simulink model "irep_single_axis"  (Simulink 7.5)
settings: Solver=ode3  StartTime=0.0  StopTime=inf  FixedStep=dt  RelTol=1e-3
InitFcn:
  | IREPOLD_DEPENDENCY
  | init_omni
  | init_filters
  | init_invivo
  | init_telemanipulation
  | init_parker_xyz
  | init_magnetic_tracker
  | init_loadcell
  | init_scopes
  | init_homing
  | init_force_control
  | ATI_Init_nano17
undefined symbols (not defined in the file): A, ATI_torque_convert_to_Nmm, counter_offset, DiscIntNeverNeededParam, dt, encoder_counts, filter_coeffs_ATI, filter_coeffs_ATI_bias, gear_ratio, HomingFineEps, HomingRoughEps, HomingRoughVelocity, inv_T, joystick_filter_coeffs, K_d, K_i, K_p, left_arm_home_voltage, N_ATI, N_ATI_bias, N_joystick, N_pots, pots_filter_coeffs, quadrature_mode, right_arm_home_voltage, RightArmHomingDirectionVector, RightArmHomingIntGain, screw_pitch
libraries: xpcconteclib x23, xpcmeasurementcomputinglib x17, xpclib x11, simulink x8, dspswit3 x4, dspsigops x1, powerlib_extras x1
(part 1 of 3)
settings Model: Creator=Andrea  LastModifiedBy=Long  BufferReuse=off
settings OptimizationCC: BlockReduction=off  OptimizeBlockIOStorage=off  BufferReuse=off  ExpressionFolding=off  LocalBlockOutputs=off  OptimizeModelRefInitCode=on
settings DebuggingCC: MultiTaskCondExecSysMsg=warning  MultiTaskRateTransMsg=warning  StrictBusMsg=Warning
settings HardwareCC: ProdIntDivRoundTo=Zero  ProdEndianess=LittleEndian  ProdHWDeviceType=Generic->32-bit x86 compatible
settings RTWCC: SystemTargetFile=xpctargetert.tlc  TemplateMakefile=xpc_ert_tmf  Description=xPC Target (ERT)  ProcessScript=xpctargetert_make_rtw_hook  RTWCompilerOptimization=On
settings xpcTargetERTCC: TargetFcnLib=ansi_tfl_table_tmw.mat  TargetFunctionLibrary=ANSI_C  UtilityFuncGeneration=Auto  ERTMultiwordTypeDef=System defined  ERTCodeCoverageTool=None  ERTMultiwordLength=256  MultiwordLength=2048  GenerateFullHeader=on  GenerateSampleERTMain=off  GenerateTestInterfaces=off  IsPILTarget=off  ModelReferenceCompliant=on  ParMdlRefBuildCompliant=off  CompOptLevelCompliant=on  IncludeMdlTerminateFcn=on  GeneratePreprocessorConditionals=Disable all  CombineOutputUpdateFcns=off  SuppressErrorStatus=off  ERTFirstTimeCompliant=off  IncludeFileDelimiter=Auto  ERTCustomFileBanners=off  SupportAbsoluteTime=on  LogVarNameModifier=rt_  MatFileLogging=on  MultiInstanceERTCode=off  SupportNonFinite=on  SupportComplex=on  PurelyIntegerCode=off  SupportContinuousTime=on  SupportNonInlinedSFcns=on  SupportVariableSizeSignals=off  EnableShiftOperators=on  ParenthesesLevel=Nominal  PortableWordSizes=off  ModelStepFunctionPrototypeControlCompliant=off  CPPClassGenCompliant=off  AutosarCompliant=off  GenerateASAP2=off  ExtModeTransport=0  ExtModeStaticAlloc=off  ExtModeStaticAllocSize=1000000  ExtModeTesting=off  InlinedParameterPlacement=NonHierarchical  TargetOS=BareBoardExample  MultiInstanceErrorCode=Error  RateGroupingCode=on  RootIOFormat=Individual arguments  CoverageDialogOpen=off  ERTFilePackagingFormat=Modular  PreserveExpressionOrder=off  PreserveIfCondition=off  ConvertIfToSwitch=off  PreserveExternInFcnDecls=on  EnableUserReplacementTypes=off  MemSecPackage=--- None ---  MemSecDataConstants=Default  MemSecDataIO=Default  MemSecDataInternal=Default  MemSecDataParameters=Default  MemSecFuncInitTerm=Default  MemSecFuncExecute=Default  GRTInterface=on  GlobalDataDefinition=Auto  GlobalDataReference=Auto  ModuleNamingRule=Unspecified  ERTSrcFileBannerTemplate=ert_code_template.cgt  ERTHdrFileBannerTemplate=ert_code_template.cgt  ERTDataSrcFileTemplate=ert_code_template.cgt  ERTDataHdrFileTemplate=ert_code_template.cgt  ERTCustomFileTemplate=example_file_process.tlc  SignalDisplayLevel=10  ParamTuneLevel=10  InitialValueSource=Model  RTWCAPISignals=off  RTWCAPIParams=off  RTWCAPIStates=off  GenerateErtSFunction=off  RL32ModeModifier=Real-Time  ExtMode=on  ExtModeMexFile=ext_xpc  ExtModeIntrfLevel=Level2 - Open  ExtModeArmWhenConnect=off  RL32LogTETModifier=on  RL32LogBufSizeModifier=100000  RL32IRQSourceModifier=Timer  xPCIRQSourceBoard=None/Other  xPCIOIRQSlot=-1  xpcObjCom=off  xPCGenerateASAP2=off  xPCGenerateXML=off  RL32ObjectName=tg  xPCisDownloadable=off  xPCisDefaultEnv=on  xPCisModelTimeout=on  xPCModelTimeoutSecs=5  xpcDblBuff=off  xPCLoadParamSetFile=off

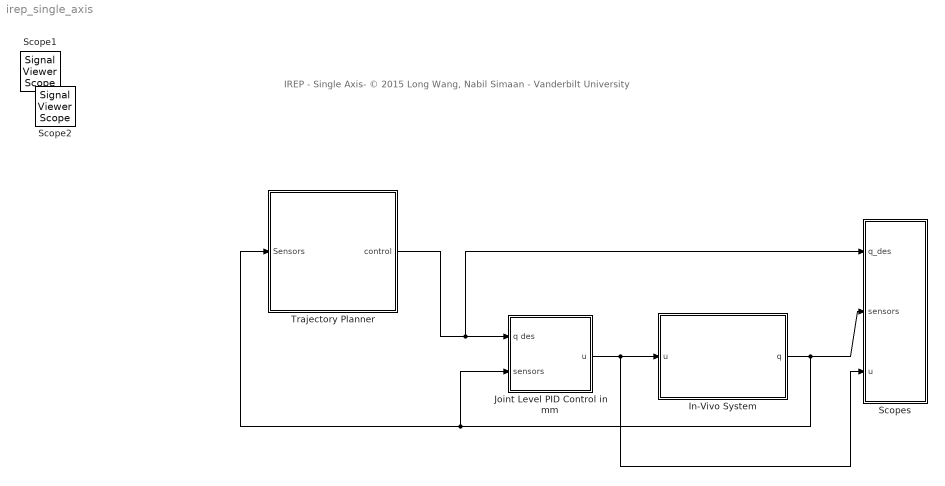
== system irep_single_axis ==
  note: IREP - Single Axis- © 2015 Long Wang, Nabil Simaan - Vanderbilt University
  In-Vivo System : Subsystem
      mask Display: image(imread('irep.png'));
  Joint Level PID Control in mm : Subsystem
  Scopes : Subsystem
  Trajectory Planner : Subsystem
  Scope1 : SignalViewerScope  IOType=viewer  RefreshTime=0.035000
  Scope2 : SignalViewerScope  IOType=viewer  RefreshTime=0.035000
  wires:
  In-Vivo System/1(q) -> Joint Level PID Control in mm/2(sensors), Trajectory Planner/1(Sensors), Scopes/2(sensors)
  Joint Level PID Control in mm/1(u) -> In-Vivo System/1(u), Scopes/3(u)
  Trajectory Planner/1(control) -> Joint Level PID Control in mm/1(q des), Scopes/1(q_des)

== system irep_single_axis/In-Vivo System ==
  u : Inport  OutDataType=fixdt(1, 16)  OutScaling=2^0
  ATI FT Sensor : Subsystem
  ATI FT Sensor enable : Constant  Value=0  OutDataType=fixdt(1, 16)  OutScaling=2^0
  Bus Creator : BusCreator  Inputs=5
  CONTEC CARDS : Subsystem
  Count to mm : Subsystem
  D/A : Subsystem
  Digital_Inputs : Subsystem
  Motor Enable : Subsystem
  Potentiometers : Subsystem
  q : Outport
  wires:
  CONTEC CARDS/1(Out1) -> Count to mm/1(counts)
  u/1 -> D/A/1(In1)
  Potentiometers/1(Pots) -> Bus Creator/2  "A/D signals"
  Bus Creator/1 -> q/1
  Count to mm/1(q_cur_system) -> Bus Creator/1  "q"
  Digital_Inputs/1(foot switches) -> Bus Creator/3  "foot switches"
  Digital_Inputs/2(Pot_connect) -> Bus Creator/4  "Pots_Connect"
  ATI FT Sensor/1(Forces) -> Bus Creator/5  "ATI"
  ATI FT Sensor enable/1 -> ATI FT Sensor/Enable

== system irep_single_axis/Joint Level PID Control in mm ==
  q des : Inport  OutDataType=fixdt(1, 16)  OutScaling=2^0
  sensors : Inport  Port=2  OutDataType=fixdt(1, 16)  OutScaling=2^0
  Bus Creator : Subsystem
  Bus selector : Subsystem
  Enable Control : Constant  Value=0  OutDataType=fixdt(1, 16)  OutScaling=2^0
  PID Compensator : Subsystem
  Sum : Sum  Inputs=|+-  OutDataType=fixdt(1, 16)  OutScaling=2^0  SampleTime=dt
  u : Outport  OutDataType=fixdt(1, 16)  OutScaling=2^0
  wires:
  q des/1 -> Sum/1
  Sum/1 -> PID Compensator/1(e)
  sensors/1 -> Bus selector/1(sensors)
  Bus selector/1(Out1) -> Sum/2
  PID Compensator/1(u) -> Bus Creator/1(In1)
  Bus Creator/1(Out1) -> u/1
  Enable Control/1 -> PID Compensator/Enable

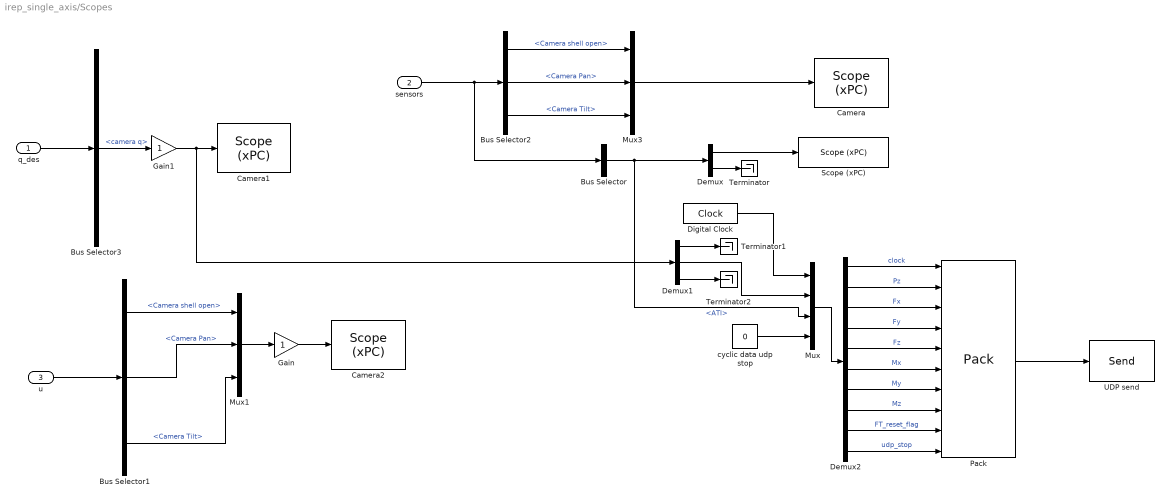
== system irep_single_axis/Scopes ==
  q_des : Inport
  sensors : Inport  Port=2
  u : Inport  Port=3
  Bus Selector : BusSelector  OutputSignals=ATI
  Bus Selector1 : BusSelector  OutputSignals=Camera shell open,Camera Pan,Camera Tilt
  Bus Selector2 : BusSelector  OutputSignals=q.Camera shell open,q.Camera Pan,q.Camera Tilt
  Bus Selector3 : BusSelector  OutputSignals=camera q
  Camera : xpclib/Misc./Scope (xPC)   SystemSampleTime=-1  scopeno=1  scopetype=Target  autostart=on  viewmode=Numerical  formatstr='Camera cur: %3.3f'  grid=on  ylimits=[0,0]  nosamples=10  noprepostsamples=0  interleave=1  triggermode=FreeRun  triggersignal=1  triggerlevel=0.0  triggerslope=Either  triggerscope=1  triggersample=0  filename=weights1.dat  mode=Lazy  writesize=512  autorestart=off  dynamicfilemode=off  maxwritefilesize=512*1024^2
  Camera1 : xpclib/Misc./Scope (xPC)   SystemSampleTime=-1  scopeno=2  scopetype=Target  autostart=on  viewmode=Numerical  formatstr='Camera des: %3.3f'  grid=on  ylimits=[0,0]  nosamples=10  noprepostsamples=0  interleave=1  triggermode=FreeRun  triggersignal=1  triggerlevel=0.0  triggerslope=Either  triggerscope=1  triggersample=0  filename=weights1.dat  mode=Lazy  writesize=512  autorestart=off  dynamicfilemode=off  maxwritefilesize=512*1024^2
  Camera2 : xpclib/Misc./Scope (xPC)   SystemSampleTime=-1  scopeno=3  scopetype=Target  autostart=on  viewmode=Numerical  formatstr='Camera u: %3.3f'  grid=on  ylimits=[0,0]  nosamples=10  noprepostsamples=0  interleave=1  triggermode=FreeRun  triggersignal=1  triggerlevel=0.0  triggerslope=Either  triggerscope=1  triggersample=0  filename=weights1.dat  mode=Lazy  writesize=512  autorestart=off  dynamicfilemode=off  maxwritefilesize=512*1024^2
  Demux : Demux  Outputs=[6,1]
  Demux1 : Demux  Outputs=3
  Demux2 : Demux  Outputs=10
  Digital Clock : DigitalClock  SampleTime=dt
  Gain : Gain  ParameterDataType=fixdt(1, 16)  ParameterScaling=2^0  OutDataType=fixdt(1, 16)  OutScaling=2^0
  Gain1 : Gain  ParameterDataType=fixdt(1, 16)  ParameterScaling=2^0  OutDataType=fixdt(1, 16)  OutScaling=2^0
  Mux : Mux
  Mux1 : Mux  Inputs=3
  Mux3 : Mux  Inputs=3
  "Pack " : xpclib/UDP/Pack  datatypes={'double' 'double' 'double' 'double' 'double' 'double' 'double' 'double' 'double' 'double'}  byteAlign=1
  "Scope (xPC) " : xpclib/Misc./Scope (xPC)   SystemSampleTime=-1  scopeno=20  scopetype=Target  autostart=on  viewmode=Numerical  formatstr=scope_format_ATI_wrench  grid=on  ylimits=[0,0]  nosamples=25  noprepostsamples=0  interleave=1  triggermode=FreeRun  triggersignal=1  triggerlevel=0.0  triggerslope=Either  triggerscope=1  triggersample=0  filename=data.dat  mode=Lazy  writesize=512  autorestart=off  dynamicfilemode=off  maxwritefilesize=512*1024^2
  Terminator : Terminator
  Terminator1 : Terminator
  Terminator2 : Terminator
  UDP send : xpclib/UDP/Send  ipAddress=192.168.1.101  ipPort=25001  localPort=-1  vblLen=off  sampletime=0.008
  cyclic data udp stop : Constant  Value=0  OutDataType=fixdt(1, 16)  OutScaling=2^0
  wires:
  sensors/1 -> Bus Selector/1, Bus Selector2/1
  q_des/1 -> Bus Selector3/1
  Bus Selector3/1 -> Gain1/1  "<camera q>"
  Mux3/1 -> Camera/1
  Bus Selector2/1 -> Mux3/1  "<Camera shell open>"
  Bus Selector2/2 -> Mux3/2  "<Camera Pan>"
  Bus Selector2/3 -> Mux3/3  "<Camera Tilt>"
  u/1 -> Bus Selector1/1
  Bus Selector1/1 -> Mux1/1  "<Camera shell open>"
  Bus Selector1/2 -> Mux1/2  "<Camera Pan>"
  Bus Selector1/3 -> Mux1/3  "<Camera Tilt>"
  Mux1/1 -> Gain/1
  Gain/1 -> Camera2/1
  Gain1/1 -> Camera1/1, Demux1/1
  Bus Selector/1 -> Demux/1, Mux/3  "<ATI>"
  Demux/1 -> "Scope (xPC) "/1
  Demux/2 -> Terminator/1
  Demux1/1 -> Terminator1/1
  Demux1/3 -> Terminator2/1
  Digital Clock/1 -> Mux/1
  Demux1/2 -> Mux/2
  Mux/1 -> Demux2/1
  Demux2/1 -> "Pack "/1  "clock"
  Demux2/2 -> "Pack "/2  "Pz"
  Demux2/3 -> "Pack "/3  "Fx"
  Demux2/4 -> "Pack "/4  "Fy"
  Demux2/5 -> "Pack "/5  "Fz"
  Demux2/6 -> "Pack "/6  "Mx"
  Demux2/7 -> "Pack "/7  "My"
  Demux2/8 -> "Pack "/8  "Mz"
  Demux2/9 -> "Pack "/9  "FT_reset_flag"
  "Pack "/1 -> UDP send/1
  cyclic data udp stop/1 -> Mux/4
  Demux2/10 -> "Pack "/10  "udp_stop"

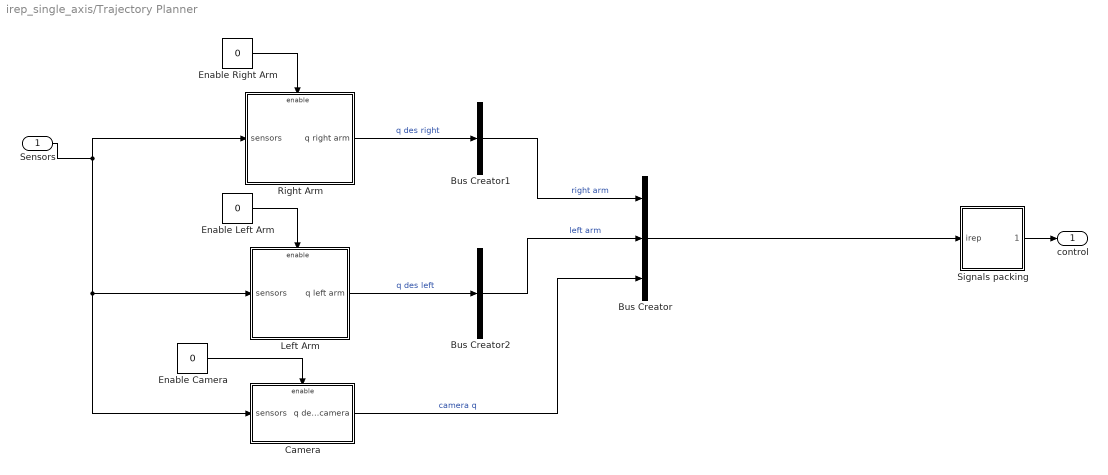
== system irep_single_axis/Trajectory Planner ==
  Sensors : Inport
  Bus Creator : BusCreator  Inputs=3
  Bus Creator1 : BusCreator  Inputs=1
  Bus Creator2 : BusCreator  Inputs=1
  Camera : Subsystem  TreatAsAtomicUnit=on
  Enable Camera : Constant  Value=0  OutDataType=fixdt(1, 16)  OutScaling=2^0  SampleTime=dt
  Enable Left Arm : Constant  Value=0  OutDataType=fixdt(1, 16)  OutScaling=2^0  SampleTime=dt
  Enable Right Arm : Constant  Value=0  OutDataType=fixdt(1, 16)  OutScaling=2^0  SampleTime=dt
  Left Arm : Subsystem  TreatAsAtomicUnit=on
  Right Arm : Subsystem  TreatAsAtomicUnit=on
  Signals packing : Subsystem
  control : Outport  PortDimensions=[23 1]  SampleTime=dt
  wires:
  Enable Right Arm/1 -> Right Arm/Enable
  Enable Left Arm/1 -> Left Arm/Enable
  Enable Camera/1 -> Camera/Enable
  Signals packing/1(system) -> control/1
  Sensors/1 -> Right Arm/1(sensors), Left Arm/1(sensors), Camera/1(sensors)
  Right Arm/1(q right arm) -> Bus Creator1/1  "q des right"
  Bus Creator1/1 -> Bus Creator/1  "right arm"
  Bus Creator2/1 -> Bus Creator/2  "left arm"
  Camera/1(q des camera) -> Bus Creator/3  "camera q"
  Bus Creator/1 -> Signals packing/1(irep)
  Left Arm/1(q left arm) -> Bus Creator2/1  "q des left"

== system irep_single_axis/In-Vivo System/ATI FT Sensor ==
  Enable : EnablePort
  ATI FT Sensor - 20001 : xpclib/UDP/Receive  ipAddress=0.0.0.0  ipPort=20001  width=48  vblLen=on  sampletime=2*dt
  ATI Force Torque Sensor : Subsystem
  Demux : Demux  Outputs=6
  Multiport Switch : MultiPortSwitch  DataPortOrder=Zero-based contiguous  Inputs=2  zeroidx=on  OutDataType=fixdt(1, 16)  OutScaling=2^0
  Mux : Mux  Inputs=7
  Mux1 : Mux  Inputs=6
  Rate Transition : RateTransition  OutPortSampleTime=dt
  Terminator1 : Terminator
  Unpack 2 : xpclib/UDP/Unpack  dimensions={1,1,1,1,1,1}  datatypes={'double' 'double' 'double' 'double' 'double' 'double'}  byteAlign=1
  input source : Constant  OutDataType=fixdt(1, 16)  OutScaling=2^0
  Forces : Outport
  wires:
  ATI FT Sensor - 20001/1 -> Unpack 2/1
  ATI FT Sensor - 20001/2 -> Terminator1/1
  Unpack 2/2 -> Mux1/2  "Fy"
  Unpack 2/3 -> Mux1/3  "Fz"
  Unpack 2/4 -> Mux1/4  "Mx"
  Unpack 2/5 -> Mux1/5  "My"
  Unpack 2/6 -> Mux1/6  "Mz"
  Unpack 2/1 -> Mux1/1  "Fx"
  Mux1/1 -> Rate Transition/1
  ATI Force Torque Sensor/1(wrench) -> Multiport Switch/3
  input source/1 -> Multiport Switch/1
  Demux/1 -> Mux/1  "Fx"
  Demux/2 -> Mux/2  "Fy"
  Demux/3 -> Mux/3  "Fz"
  Demux/4 -> Mux/4  "Mx"
  Demux/5 -> Mux/5  "My"
  Demux/6 -> Mux/6  "Mz"
  Multiport Switch/1 -> Demux/1
  Mux/1 -> Forces/1
  Rate Transition/1 -> Multiport Switch/2
  ATI Force Torque Sensor/2(reset flag) -> Mux/7  "FT_Reset_Flag"

== system irep_single_axis/In-Vivo System/CONTEC CARDS ==
  Level 1 : Subsystem
  Level 2 : Subsystem
  Level 3 : Subsystem
  Mux : Mux
  RZ : Subsystem
  Out1 : Outport
  wires:
  Level 1/1(Out1) -> Mux/1
  Level 2/1(Out1) -> Mux/2
  Level 3/1(Out1) -> Mux/3
  Mux/1 -> Out1/1
  RZ/1(Out1) -> Mux/4

== system irep_single_axis/In-Vivo System/Count to mm ==
  counts : Inport  OutDataType=sfix(16)  OutScaling=2^0
  Bus Creator : Subsystem
  Subtract : Sum  Inputs=+-  OutDataType=sfix(16)  OutScaling=2^-10
  counter_offset : Constant  Value=counter_offset*ones(23,1)  OutDataType=sfix(16)  OutScaling=2^0  SampleTime=dt
  counts  to mm : Gain  Gain=screw_pitch./(quadrature_mode*encoder_counts.*gear_ratio)  ParameterDataType=sfix(16)  ParameterScaling=2^0  OutDataType=sfix(16)  OutScaling=2^0  SampleTime=dt
  q_cur_system : Outport  OutDataType=sfix(16)  OutScaling=2^0
  wires:
  Subtract/1 -> counts  to mm/1
  counter_offset/1 -> Subtract/2
  counts/1 -> Subtract/1
  Bus Creator/1(Out1) -> q_cur_system/1
  counts  to mm/1 -> Bus Creator/1(In1)

== system irep_single_axis/In-Vivo System/D/A ==
  In1 : Inport
  Bus Selector : BusSelector  OutputSignals=Parker insertion stage,Parker rotary stage
  Bus Selector 1 : Subsystem
  Bus Selector 2 : Subsystem
  Bus Selector 3 : Subsystem
  Gain : Gain  Gain=-1  ParameterDataType=fixdt(1, 16)  ParameterScaling=2^0  OutDataType=fixdt(1, 16)  OutScaling=2^0
  Gain1 : Gain  Gain=-1  ParameterDataType=fixdt(1, 16)  ParameterScaling=2^0  OutDataType=fixdt(1, 16)  OutScaling=2^0
  Level 1 : Subsystem
  Level 2 : Subsystem
  Level 3 : Subsystem
  "PCI-DAS1602 12 " : xpcmeasurementcomputinglib/D//A/PCI-DAS1602 12   channel=[1 2]  range=[-10 -10]  reset=[1 1]  initValue=[0 0]  sampletime=dt  pci_dev=[1 14]
  wires:
  Bus Selector 1/1(Out1) -> Level 1/1(In1)
  Bus Selector 2/1(Out1) -> Level 2/1(In1)
  Bus Selector 3/1(Out1) -> Level 3/1(In1)
  In1/1 -> Bus Selector 2/1(In1), Bus Selector 1/1(In1), Bus Selector 3/1(In1), Bus Selector/1
  Bus Selector/2 -> Gain/1  "<Parker rotary stage>"
  Bus Selector/1 -> Gain1/1  "<Parker insertion stage>"
  Gain/1 -> "PCI-DAS1602 12 "/2
  Gain1/1 -> "PCI-DAS1602 12 "/1

== system irep_single_axis/In-Vivo System/Digital_Inputs ==
  Bus Creator1 : BusCreator  Inputs=2
  Bus Creator2 : BusCreator  Inputs=2
  Left Pot Front connect : xpcmeasurementcomputinglib/Digital Input/PCI-DAS1602 12   channel=[5]  port=B  chip=1  sampletime=dt  slot=[2 9]
  Left Pot Rear connect : xpcmeasurementcomputinglib/Digital Input/PCI-DAS1602 12   channel=[6]  port=B  chip=1  sampletime=dt  slot=[2 9]
  Left foot switch : xpcmeasurementcomputinglib/Digital Input/PCI-DAS1602 12   channel=[1]  port=B  chip=1  sampletime=dt  slot=[2 9]
  Mux : Mux  Inputs=2
  Mux1 : Mux  Inputs=2
  Righ foot switch : xpcmeasurementcomputinglib/Digital Input/PCI-DAS1602 12   channel=[2]  port=B  chip=1  sampletime=dt  slot=[2 9]
  Right Pot Front connect : xpcmeasurementcomputinglib/Digital Input/PCI-DAS1602 12   channel=[3]  port=B  chip=1  sampletime=dt  slot=[2 9]
  Right Pot Rear connect : xpcmeasurementcomputinglib/Digital Input/PCI-DAS1602 12   channel=[4]  port=B  chip=1  sampletime=dt  slot=[2 9]
  foot switches : Outport
  Pot_connect : Outport  Port=2
  wires:
  Left foot switch/1 -> Bus Creator1/2  "left foot switch"
  Righ foot switch/1 -> Bus Creator1/1  "right foot switch"
  Bus Creator1/1 -> foot switches/1
  Bus Creator2/1 -> Pot_connect/1
  Right Pot Front connect/1 -> Mux/1
  Right Pot Rear connect/1 -> Mux/2
  Left Pot Front connect/1 -> Mux1/1
  Left Pot Rear connect/1 -> Mux1/2
  Mux/1 -> Bus Creator2/1  "R_Pots_Connect"
  Mux1/1 -> Bus Creator2/2  "L_Pots_Connect"

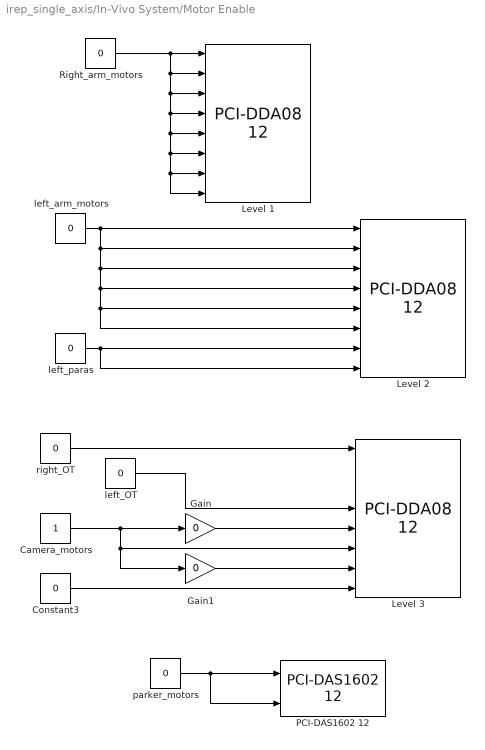
== system irep_single_axis/In-Vivo System/Motor Enable ==
  Camera_motors : Constant  OutDataType=fixdt(1, 16)  OutScaling=2^0
  Constant3 : Constant  Value=0  OutDataType=fixdt(1, 16)  OutScaling=2^0
  Gain : Gain  Gain=0  ParameterDataType=fixdt(1, 16)  ParameterScaling=2^0  OutDataType=fixdt(1, 16)  OutScaling=2^0
  Gain1 : Gain  Gain=0  ParameterDataType=fixdt(1, 16)  ParameterScaling=2^0  OutDataType=fixdt(1, 16)  OutScaling=2^0
  Level 1 : xpcmeasurementcomputinglib/Digital Output/PCI-DDA08 12   channel=[1 2 3 4 5 6 7 8]  port=C  reset=[1 1 1 1 1 1 1 1]  initValue=[0 0 0 0 0 0 0 0]  chip=1  sampletime=dt  slot=[2, 7]
  Level 2 : xpcmeasurementcomputinglib/Digital Output/PCI-DDA08 12   channel=[1 2 3 4 5 6 7 8]  port=C  reset=[1 1 1 1 1 1 1 1]  initValue=[0 0 0 0 0 0 0 0]  chip=1  sampletime=dt  slot=[2, 10]
  Level 3 : xpcmeasurementcomputinglib/Digital Output/PCI-DDA08 12   channel=[1 2 3 4 5 6 7 8]  port=C  reset=[1 1 1 1 1 1 1 1]  initValue=[0 0 0 0 0 0 0 0]  chip=1  sampletime=dt  slot=[2, 13]
  "PCI-DAS1602 12 " : xpcmeasurementcomputinglib/Digital Output/PCI-DAS1602 12   channel=[1 2]  port=A  reset=[1 1]  initValue=[0 0]  chip=1  sampletime=dt  slot=[2 9]
  Right_arm_motors : Constant  Value=0  OutDataType=fixdt(1, 16)  OutScaling=2^0
  left_OT : Constant  Value=0  OutDataType=fixdt(1, 16)  OutScaling=2^0
  left_arm_motors : Constant  Value=0  OutDataType=fixdt(1, 16)  OutScaling=2^0
  left_paras : Constant  Value=0  OutDataType=fixdt(1, 16)  OutScaling=2^0
  parker_motors : Constant  Value=0  OutDataType=fixdt(1, 16)  OutScaling=2^0
  right_OT : Constant  Value=0  OutDataType=fixdt(1, 16)  OutScaling=2^0
  wires:
  Right_arm_motors/1 -> Level 1/1, Level 1/2, Level 1/3, Level 1/4, Level 1/5, Level 1/6, Level 1/7, Level 1/8
  left_arm_motors/1 -> Level 2/1, Level 2/2, Level 2/3, Level 2/4, Level 2/5, Level 2/6
  Camera_motors/1 -> Level 3/6, Gain1/1, Gain/1
  Constant3/1 -> Level 3/8
  left_paras/1 -> Level 2/7, Level 2/8
  parker_motors/1 -> "PCI-DAS1602 12 "/1, "PCI-DAS1602 12 "/2
  right_OT/1 -> Level 3/1
  left_OT/1 -> Level 3/4
  Gain/1 -> Level 3/5
  Gain1/1 -> Level 3/7

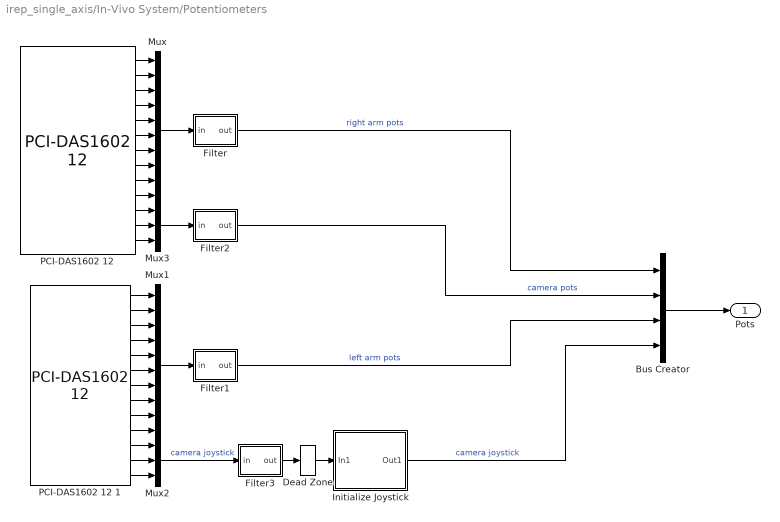
== system irep_single_axis/In-Vivo System/Potentiometers ==
  Bus Creator : BusCreator
  Dead Zone : DeadZone  LowerValue=2.5-0.4  UpperValue=2.5+0.4  SaturateOnIntegerOverflow=on
  Filter : Subsystem
  Filter1 : Subsystem
  Filter2 : Subsystem
  Filter3 : Subsystem
  Initialize Joystick : Subsystem
  Mux : Mux  Inputs=10
  Mux1 : Mux  Inputs=10
  Mux2 : Mux  Inputs=3
  Mux3 : Mux  Inputs=3
  "PCI-DAS1602 12 " : xpcmeasurementcomputinglib/A//D/PCI-DAS1602 12   channel=13  range=+-5V  mux=Single-ended (16 channels)  sampletime=dt  slot=[1 14]
  PCI-DAS1602 12 1 : xpcmeasurementcomputinglib/A//D/PCI-DAS1602 12   channel=13  range=+-5V  mux=Single-ended (16 channels)  sampletime=dt  slot=[2 9]
  Pots : Outport
  wires:
  "PCI-DAS1602 12 "/1 -> Mux/1
  "PCI-DAS1602 12 "/2 -> Mux/2
  "PCI-DAS1602 12 "/3 -> Mux/3
  "PCI-DAS1602 12 "/4 -> Mux/4
  "PCI-DAS1602 12 "/5 -> Mux/5
  "PCI-DAS1602 12 "/6 -> Mux/6
  "PCI-DAS1602 12 "/7 -> Mux/7
  "PCI-DAS1602 12 "/8 -> Mux/8
  "PCI-DAS1602 12 "/9 -> Mux/9
  "PCI-DAS1602 12 "/10 -> Mux/10
  PCI-DAS1602 12 1/11 -> Mux2/1
  PCI-DAS1602 12 1/10 -> Mux1/10
  PCI-DAS1602 12 1/9 -> Mux1/9
  PCI-DAS1602 12 1/8 -> Mux1/8
  PCI-DAS1602 12 1/7 -> Mux1/7
  PCI-DAS1602 12 1/6 -> Mux1/6
  PCI-DAS1602 12 1/5 -> Mux1/5
  PCI-DAS1602 12 1/4 -> Mux1/4
  PCI-DAS1602 12 1/3 -> Mux1/3
  PCI-DAS1602 12 1/2 -> Mux1/2
  PCI-DAS1602 12 1/1 -> Mux1/1
  Bus Creator/1 -> Pots/1
  Mux/1 -> Filter/1(in)
  Filter1/1(out) -> Bus Creator/3  "left arm pots"
  Mux1/1 -> Filter1/1(in)
  PCI-DAS1602 12 1/12 -> Mux2/2
  PCI-DAS1602 12 1/13 -> Mux2/3
  Mux2/1 -> Filter3/1(in)  "camera joystick"
  "PCI-DAS1602 12 "/12 -> Mux3/2
  "PCI-DAS1602 12 "/13 -> Mux3/3
  "PCI-DAS1602 12 "/11 -> Mux3/1
  Initialize Joystick/1(Out1) -> Bus Creator/4  "camera joystick"
  Filter/1(out) -> Bus Creator/1  "right arm pots"
  Mux3/1 -> Filter2/1(in)
  Filter2/1(out) -> Bus Creator/2  "camera pots"
  Dead Zone/1 -> Initialize Joystick/1(In1)
  Filter3/1(out) -> Dead Zone/1

== system irep_single_axis/Joint Level PID Control in mm/Bus Creator ==
  In1 : Inport
  Bus Creator : BusCreator  Inputs=23
  Demux : Demux  Outputs=23
  Out1 : Outport
  wires:
  Demux/1 -> Bus Creator/1  "Righ arm - Overall Translational Movement"
  Demux/2 -> Bus Creator/2  "Right arm - Parallelogram Insert"
  Demux/3 -> Bus Creator/3  "Right arm - Parallelogram Deploy"
  Demux/4 -> Bus Creator/4  "Right arm - Proximal Segment X"
  Demux/5 -> Bus Creator/5  "Right arm - Proximal Segment Y"
  Demux/6 -> Bus Creator/6  "Right arm - Distal Segment X"
  Demux/7 -> Bus Creator/7  "Right arm - Distal Segment Y"
  Demux/8 -> Bus Creator/8  "Right arm - Wrist Joint"
  Demux/9 -> Bus Creator/9  "Right arm - Gripper Joint"
  Demux/10 -> Bus Creator/10  "Left arm - Overall Translational Movement"
  Demux/11 -> Bus Creator/11  "Left arm - Parallelogram Insert"
  Demux/12 -> Bus Creator/12  "Left arm - Parallelogram Deploy"
  Demux/13 -> Bus Creator/13  "Left arm - Proximal Segment X"
  Demux/14 -> Bus Creator/14  "Left arm - Proximal Segment Y"
  Demux/15 -> Bus Creator/15  "Left arm - Distal Segment X"
  Demux/16 -> Bus Creator/16  "Left arm - Distal Segment Y"
  Demux/17 -> Bus Creator/17  "Left arm - Wrist Joint"
  Demux/18 -> Bus Creator/18  "Left arm - Gripper Joint"
  Demux/19 -> Bus Creator/19  "Camera shell open"
  Demux/20 -> Bus Creator/20  "Camera Pan"
  Demux/21 -> Bus Creator/21  "Camera Tilt"
  Bus Creator/1 -> Out1/1
  In1/1 -> Demux/1
  Demux/22 -> Bus Creator/22  "Parker insertion stage"
  Demux/23 -> Bus Creator/23  "Parker rotary stage"

== system irep_single_axis/Joint Level PID Control in mm/Bus selector ==
  sensors : Inport
  Camera selector : Subsystem
  Left arm selector : Subsystem
  Mux : Mux
  RZ : Subsystem
  Right arm  selector : Subsystem
  Out1 : Outport
  wires:
  Left arm selector/1(Out1) -> Mux/2
  Right arm  selector/1(Out1) -> Mux/1
  Camera selector/1(Out1) -> Mux/3
  Mux/1 -> Out1/1
  sensors/1 -> Left arm selector/1(In1), Right arm  selector/1(In1), Camera selector/1(In1), RZ/1(In1)
  RZ/1(Out1) -> Mux/4

== system irep_single_axis/Joint Level PID Control in mm/PID Compensator ==
  e : Inport  OutDataType=sfix(16)  OutScaling=2^0
  Enable : EnablePort
  Add : Sum  Inputs=+++  OutDataType=sfix(16)  OutScaling=2^-10
  Discrete Derivative : simulink/Discrete/Discrete Derivative  SystemSampleTime=-1  gainval=1.0  ICPrevScaledInput=0.0  OutMin=[]  OutMax=[]  OutDataType=sfix(16)  OutScaling=2^-10  DoSatur=off
  Discrete-Time Integrator : DiscreteIntegrator  SampleTime=dt  OutDataType=sfix(16)  OutScaling=2^0  ICPrevOutput=DiscIntNeverNeededParam  ICPrevScaledInput=DiscIntNeverNeededParam
  Integral Sat : Saturate  UpperLimit=5  LowerLimit=-5  OutDataType=sfix(16)  OutScaling=2^0
  Kd : Gain  Gain=K_d  ParameterDataType=sfix(16)  ParameterScaling=2^0  OutDataType=sfix(16)  OutScaling=2^0  SampleTime=dt
  Ki : Gain  Gain=K_i  ParameterDataType=sfix(16)  ParameterScaling=2^0  OutDataType=sfix(16)  OutScaling=2^0  SampleTime=dt
  Kp : Gain  Gain=K_p  ParameterDataType=sfix(16)  ParameterScaling=2^0  OutDataType=sfix(16)  OutScaling=2^0  SampleTime=dt
  Saturation : Saturate  UpperLimit=10  LowerLimit=-10  OutDataType=sfix(16)  OutScaling=2^0
  u : Outport  OutDataType=sfix(16)  OutScaling=2^0  InitialOutput=zeros(23,1)
  wires:
  Discrete Derivative/1 -> Add/3
  Kd/1 -> Discrete Derivative/1
  Integral Sat/1 -> Add/2
  Discrete-Time Integrator/1 -> Integral Sat/1
  Saturation/1 -> u/1
  Add/1 -> Saturation/1
  Ki/1 -> Discrete-Time Integrator/1
  Kp/1 -> Add/1
  e/1 -> Ki/1, Kp/1, Kd/1

== system irep_single_axis/Trajectory Planner/Camera ==
  sensors : Inport  OutDataType=fixdt(1, 16)  OutScaling=2^0
  Enable : EnablePort
  Bus Selector : BusSelector  OutputSignals=ATI.FT_Reset_Flag
  Contact Detection : Subsystem
  Enable Joint Space : Constant  Value=0  OutDataType=fixdt(1, 16)  OutScaling=2^0  SampleTime=dt
  Joint Space : Subsystem  TreatAsAtomicUnit=on
  Mux : Mux  Inputs=[2,1]
  "Scope (xPC) " : xpclib/Misc./Scope (xPC)   SystemSampleTime=-1  scopeno=4  scopetype=Target  autostart=on  viewmode=Numerical  formatstr='c %15.6f'  grid=on  ylimits=[0,0]  nosamples=10  noprepostsamples=0  interleave=1  triggermode=FreeRun  triggersignal=1  triggerlevel=0.0  triggerslope=Either  triggerscope=1  triggersample=0  filename=data.dat  mode=Lazy  writesize=512  autorestart=off  dynamicfilemode=off  maxwritefilesize=512*1024^2
  Terminator : Terminator
  q des camera : Outport  OutDataType=fixdt(1, 16)  OutScaling=2^0  InitialOutput=zeros(3,1)
  wires:
  Enable Joint Space/1 -> Joint Space/Enable
  Joint Space/1(Out1) -> q des camera/1
  sensors/1 -> Joint Space/1(sensors), Contact Detection/1(sensors), Bus Selector/1
  Contact Detection/1(c) -> Terminator/1, Mux/1
  Bus Selector/1 -> Mux/2  "<FT_Reset_Flag>"
  Mux/1 -> "Scope (xPC) "/1

== system irep_single_axis/Trajectory Planner/Left Arm ==
  note: IREP Left Arm Trajectory Planner - v 0.6 - © COPYRIGHT 2011 Andrea Bajo, Nabil Simaan
  sensors : Inport  OutDataType=fixdt(1, 16)  OutScaling=2^0
  Enable : EnablePort
  Enable Low Level : Constant  Value=0  OutDataType=fixdt(1, 16)  OutScaling=2^0  SampleTime=dt
  Low Level : Subsystem  TreatAsAtomicUnit=on
  q left arm : Outport  OutDataType=fixdt(1, 16)  OutScaling=2^0  InitialOutput=zeros(9,1)
  wires:
  Enable Low Level/1 -> Low Level/Enable
  Low Level/1(q des) -> q left arm/1
  sensors/1 -> Low Level/1(sensors)

== system irep_single_axis/Trajectory Planner/Right Arm ==
  note: IREP Right Arm Trajectory Planner - v 1.0 - © COPYRIGHT 2011 Andrea Bajo, Nabil Simaan
  sensors : Inport  OutDataType=fixdt(1, 16)  OutScaling=2^0
  Enable : EnablePort
  Enable Low Level : Constant  Value=0  OutDataType=fixdt(1, 16)  OutScaling=2^0  SampleTime=dt
  Low Level : Subsystem  TreatAsAtomicUnit=on
  q right arm : Outport  OutDataType=fixdt(1, 16)  OutScaling=2^0  InitialOutput=zeros(9,1)
  wires:
  Enable Low Level/1 -> Low Level/Enable
  Low Level/1(q des) -> q right arm/1
  sensors/1 -> Low Level/1(sensors)

== system irep_single_axis/Trajectory Planner/Signals packing ==
  irep : Inport
  Bus Selector : BusSelector  OutputSignals=right arm.q des right,left arm.q des left,camera q
  Constant : Constant  Value=zeros(2,1)  OutDataType=fixdt(1, 16)  OutScaling=2^0
  Mux : Mux
  system : Outport
  wires:
  Bus Selector/1 -> Mux/1  "<q des right>"
  Bus Selector/2 -> Mux/2  "<q des left>"
  Bus Selector/3 -> Mux/3  "<camera q>"
  irep/1 -> Bus Selector/1
  Mux/1 -> system/1
  Constant/1 -> Mux/4

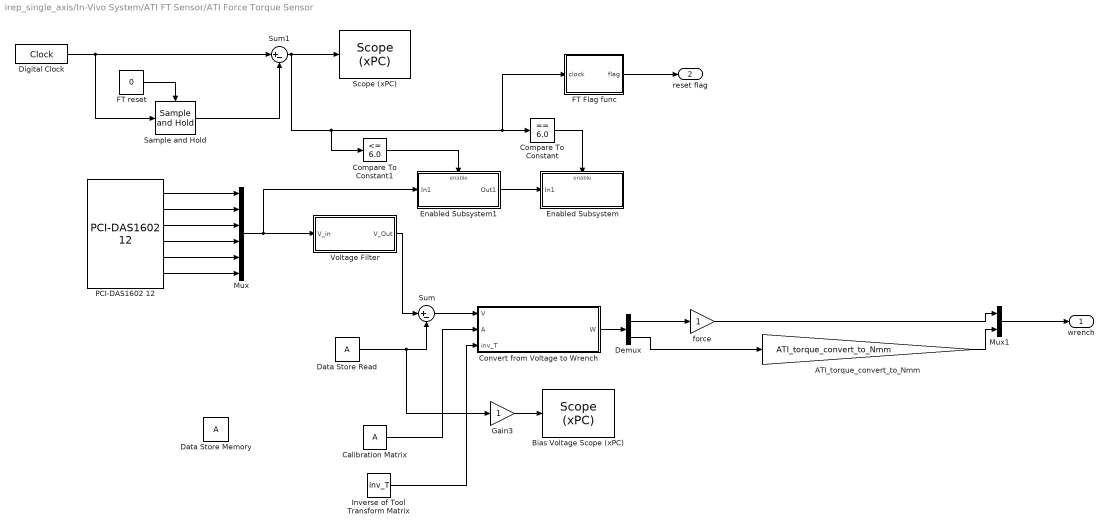
== system irep_single_axis/In-Vivo System/ATI FT Sensor/ATI Force Torque Sensor ==
  ATI_torque_convert_to_Nmm : Gain  Gain=ATI_torque_convert_to_Nmm
  Bias Voltage Scope (xPC) : xpclib/Misc./Scope (xPC)   SystemSampleTime=-1  scopeno=6  scopetype=Host  autostart=on  viewmode=Numerical  formatstr=Voltage_Vals_format  grid=on  ylimits=[0,0]  nosamples=250  noprepostsamples=0  interleave=1  triggermode=FreeRun  triggersignal=1  triggerlevel=0.0  triggerslope=Either  triggerscope=1  triggersample=0  filename=data.dat  mode=Lazy  writesize=512  autorestart=off  dynamicfilemode=off  maxwritefilesize=512*1024^2
  Calibration Matrix : Constant  Value=A
  Compare To Constant : simulink/Logic and Bit Operations/Compare To Constant  SystemSampleTime=-1  relop===  const=6.0  LogicOutDataTypeMode=uint8  ZeroCross=off
  Compare To Constant1 : simulink/Logic and Bit Operations/Compare To Constant  SystemSampleTime=-1  relop=<=  const=6.0  LogicOutDataTypeMode=uint8  ZeroCross=off
  "Convert from Voltage to Wrench " : Stateflow chart  TreatAsAtomicUnit=on
  Data Store Memory : DataStoreMemory  DataStoreName=A  ReadBeforeWriteMsg=warning  WriteAfterWriteMsg=warning  WriteAfterReadMsg=warning  InitialValue=[0;0;0;0;0;0]
  Data Store Read : DataStoreRead  DataStoreName=A  SampleTime=0
  Demux : Demux  Outputs=2
  Digital Clock : DigitalClock  SampleTime=dt
  Enabled Subsystem : Subsystem  TreatAsAtomicUnit=on
  Enabled Subsystem1 : Subsystem  TreatAsAtomicUnit=on
  FT Flag func : Stateflow chart  TreatAsAtomicUnit=on
  FT reset : Constant  Value=0  OutDataType=fixdt(1, 16)  OutScaling=2^0
  Gain3 : Gain
  Inverse of Tool Transform Matrix : Constant  Value=inv_T  VectorParams1D=off
  Mux : Mux  Inputs=6
  Mux1 : Mux  Inputs=2
  "PCI-DAS1602 12 " : xpcmeasurementcomputinglib/A//D/PCI-DAS1602 12   channel=6  range=+-10V  mux=Differential (8 channels)  sampletime=dt  slot=[2 12]
  Sample and Hold : dspsigops/Sample and Hold  SystemSampleTime=-1  trig=Rising edge  initCond=0  latchinput=off
  "Scope (xPC) " : xpclib/Misc./Scope (xPC)   SystemSampleTime=-1  scopeno=5  scopetype=Host  autostart=on  viewmode=Numerical  formatstr='%15.6f'  grid=on  ylimits=[0,0]  nosamples=25  noprepostsamples=0  interleave=1  triggermode=FreeRun  triggersignal=1  triggerlevel=0.0  triggerslope=Either  triggerscope=1  triggersample=0  filename=data.dat  mode=Lazy  writesize=512  autorestart=off  dynamicfilemode=off  maxwritefilesize=512*1024^2
  Sum : Sum  Inputs=|+-
  Sum1 : Sum  Inputs=|+-  OutDataType=fixdt(1, 16)  OutScaling=2^0
  Voltage Filter : Subsystem
  force : Gain
  wrench : Outport  OutDataType=fixdt(1, 16)  OutScaling=2^0
  reset flag : Outport  Port=2  OutDataType=fixdt(1, 16)  OutScaling=2^0
  wires:
  Mux/1 -> Voltage Filter/1(V_in), Enabled Subsystem1/1(In1)
  Calibration Matrix/1 -> "Convert from Voltage to Wrench "/2(A)
  Inverse of Tool Transform Matrix/1 -> "Convert from Voltage to Wrench "/3(inv_T)
  Sum/1 -> "Convert from Voltage to Wrench "/1(V)
  Voltage Filter/1(V_Out) -> Sum/1
  Data Store Read/1 -> Sum/2, Gain3/1
  Enabled Subsystem1/1(Out1) -> Enabled Subsystem/1(In1)
  Compare To Constant/1 -> Enabled Subsystem/Enable
  Gain3/1 -> Bias Voltage Scope (xPC)/1
  Compare To Constant1/1 -> Enabled Subsystem1/Enable
  Digital Clock/1 -> Sum1/1, Sample and Hold/1
  Sum1/1 -> Compare To Constant1/1, Compare To Constant/1, FT Flag func/1(clock), "Scope (xPC) "/1
  Sample and Hold/1 -> Sum1/2
  FT reset/1 -> Sample and Hold/Trigger
  Demux/1 -> force/1
  Demux/2 -> ATI_torque_convert_to_Nmm/1
  ATI_torque_convert_to_Nmm/1 -> Mux1/2
  force/1 -> Mux1/1
  Mux1/1 -> wrench/1
  "Convert from Voltage to Wrench "/1(W) -> Demux/1
  "PCI-DAS1602 12 "/1 -> Mux/1
  "PCI-DAS1602 12 "/2 -> Mux/2
  "PCI-DAS1602 12 "/3 -> Mux/3
  "PCI-DAS1602 12 "/4 -> Mux/4
  "PCI-DAS1602 12 "/5 -> Mux/5
  "PCI-DAS1602 12 "/6 -> Mux/6
  FT Flag func/1(flag) -> reset flag/1

== system irep_single_axis/In-Vivo System/CONTEC CARDS/Level 1 ==
  Mux : Mux  Inputs=8
  enc 1 : xpcconteclib/Incremental Encoder/CNT32-8M(PCI)   Channel=1  OperationMode=2-phase Input Synchronous Clear Multiply by 4  DigitalFilter=No filtering  PulseInput=TTL level input  Direction=Up in the clockwise direction/Down in the counterclockwise direction  InitialValue=counter_offset_init  LoadInitialValue=on  SampleTime=dt  PciSlot=[1,13]  StartMethod=Model Start  StopMethod=Model Terminate  ZeroClearRising=off  ZeroClearFalling=off  ZeroClearMatch0=off  ZeroClearMatch1=off  PresetRising=on  PresetFalling=off  PresetMatch0=off  PresetMatch1=off  PresetValue=0  Match0Value=0  Match1Value=0  OutputSignalMatch0=off  OutputSignalMatch1=off  OutputSignalAbnormal=off  OutputSignalDigitalFilter=off  OutputSignalAlarm=off  OneShotDuration=10 microseconds  IndexEnable=Disable  IndexLogic=Positive (Active High)  EnableDigitalInput=off  EnableDigitalOutput=off  DigitalOutputInitialValue=None  DigitalOutputFinalValue=None
  enc 2 : xpcconteclib/Incremental Encoder/CNT32-8M(PCI)   Channel=2  OperationMode=2-phase Input Synchronous Clear Multiply by 4  DigitalFilter=No filtering  PulseInput=TTL level input  Direction=Up in the clockwise direction/Down in the counterclockwise direction  InitialValue=counter_offset_init  LoadInitialValue=on  SampleTime=dt  PciSlot=[1,13]  StartMethod=Model Start  StopMethod=Model Terminate  ZeroClearRising=off  ZeroClearFalling=off  ZeroClearMatch0=off  ZeroClearMatch1=off  PresetRising=off  PresetFalling=off  PresetMatch0=off  PresetMatch1=off  PresetValue=0  Match0Value=0  Match1Value=0  OutputSignalMatch0=off  OutputSignalMatch1=off  OutputSignalAbnormal=off  OutputSignalDigitalFilter=off  OutputSignalAlarm=off  OneShotDuration=10 microseconds  IndexEnable=Disable  IndexLogic=Positive (Active High)  EnableDigitalInput=off  EnableDigitalOutput=off  DigitalOutputInitialValue=None  DigitalOutputFinalValue=None
  enc 3 : xpcconteclib/Incremental Encoder/CNT32-8M(PCI)   Channel=3  OperationMode=2-phase Input Synchronous Clear Multiply by 4  DigitalFilter=No filtering  PulseInput=TTL level input  Direction=Down in the clockwise direction/Up in the counterclockwise direction  InitialValue=counter_offset_init  LoadInitialValue=on  SampleTime=dt  PciSlot=[1,13]  StartMethod=Model Start  StopMethod=Model Terminate  ZeroClearRising=off  ZeroClearFalling=off  ZeroClearMatch0=off  ZeroClearMatch1=off  PresetRising=off  PresetFalling=off  PresetMatch0=off  PresetMatch1=off  PresetValue=0  Match0Value=0  Match1Value=0  OutputSignalMatch0=off  OutputSignalMatch1=off  OutputSignalAbnormal=off  OutputSignalDigitalFilter=off  OutputSignalAlarm=off  OneShotDuration=10 microseconds  IndexEnable=Disable  IndexLogic=Positive (Active High)  EnableDigitalInput=off  EnableDigitalOutput=off  DigitalOutputInitialValue=None  DigitalOutputFinalValue=None
  enc 4 : xpcconteclib/Incremental Encoder/CNT32-8M(PCI)   Channel=4  OperationMode=2-phase Input Synchronous Clear Multiply by 4  DigitalFilter=No filtering  PulseInput=TTL level input  Direction=Down in the clockwise direction/Up in the counterclockwise direction  InitialValue=counter_offset_init  LoadInitialValue=on  SampleTime=dt  PciSlot=[1,13]  StartMethod=Model Start  StopMethod=Model Terminate  ZeroClearRising=off  ZeroClearFalling=off  ZeroClearMatch0=off  ZeroClearMatch1=off  PresetRising=off  PresetFalling=off  PresetMatch0=off  PresetMatch1=off  PresetValue=0  Match0Value=0  Match1Value=0  OutputSignalMatch0=off  OutputSignalMatch1=off  OutputSignalAbnormal=off  OutputSignalDigitalFilter=off  OutputSignalAlarm=off  OneShotDuration=10 microseconds  IndexEnable=Disable  IndexLogic=Positive (Active High)  EnableDigitalInput=off  EnableDigitalOutput=off  DigitalOutputInitialValue=None  DigitalOutputFinalValue=None
  enc 5 : xpcconteclib/Incremental Encoder/CNT32-8M(PCI)   Channel=5  OperationMode=2-phase Input Synchronous Clear Multiply by 4  DigitalFilter=No filtering  PulseInput=TTL level input  Direction=Up in the clockwise direction/Down in the counterclockwise direction  InitialValue=counter_offset_init  LoadInitialValue=on  SampleTime=dt  PciSlot=[1,13]  StartMethod=Model Start  StopMethod=Model Terminate  ZeroClearRising=off  ZeroClearFalling=off  ZeroClearMatch0=off  ZeroClearMatch1=off  PresetRising=off  PresetFalling=off  PresetMatch0=off  PresetMatch1=off  PresetValue=0  Match0Value=0  Match1Value=0  OutputSignalMatch0=off  OutputSignalMatch1=off  OutputSignalAbnormal=off  OutputSignalDigitalFilter=off  OutputSignalAlarm=off  OneShotDuration=10 microseconds  IndexEnable=Disable  IndexLogic=Positive (Active High)  EnableDigitalInput=off  EnableDigitalOutput=off  DigitalOutputInitialValue=None  DigitalOutputFinalValue=None
  enc 6 : xpcconteclib/Incremental Encoder/CNT32-8M(PCI)   Channel=6  OperationMode=2-phase Input Synchronous Clear Multiply by 4  DigitalFilter=No filtering  PulseInput=TTL level input  Direction=Up in the clockwise direction/Down in the counterclockwise direction  InitialValue=counter_offset_init  LoadInitialValue=on  SampleTime=dt  PciSlot=[1,13]  StartMethod=Model Start  StopMethod=Model Terminate  ZeroClearRising=off  ZeroClearFalling=off  ZeroClearMatch0=off  ZeroClearMatch1=off  PresetRising=off  PresetFalling=off  PresetMatch0=off  PresetMatch1=off  PresetValue=0  Match0Value=0  Match1Value=0  OutputSignalMatch0=off  OutputSignalMatch1=off  OutputSignalAbnormal=off  OutputSignalDigitalFilter=off  OutputSignalAlarm=off  OneShotDuration=10 microseconds  IndexEnable=Disable  IndexLogic=Positive (Active High)  EnableDigitalInput=off  EnableDigitalOutput=off  DigitalOutputInitialValue=None  DigitalOutputFinalValue=None
  enc 7 : xpcconteclib/Incremental Encoder/CNT32-8M(PCI)   Channel=7  OperationMode=2-phase Input Synchronous Clear Multiply by 4  DigitalFilter=No filtering  PulseInput=TTL level input  Direction=Down in the clockwise direction/Up in the counterclockwise direction  InitialValue=counter_offset_init  LoadInitialValue=on  SampleTime=dt  PciSlot=[1,13]  StartMethod=Model Start  StopMethod=Model Terminate  ZeroClearRising=off  ZeroClearFalling=off  ZeroClearMatch0=off  ZeroClearMatch1=off  PresetRising=off  PresetFalling=off  PresetMatch0=off  PresetMatch1=off  PresetValue=0  Match0Value=0  Match1Value=0  OutputSignalMatch0=off  OutputSignalMatch1=off  OutputSignalAbnormal=off  OutputSignalDigitalFilter=off  OutputSignalAlarm=off  OneShotDuration=10 microseconds  IndexEnable=Disable  IndexLogic=Positive (Active High)  EnableDigitalInput=off  EnableDigitalOutput=off  DigitalOutputInitialValue=None  DigitalOutputFinalValue=None
  enc 8 : xpcconteclib/Incremental Encoder/CNT32-8M(PCI)   Channel=8  OperationMode=2-phase Input Synchronous Clear Multiply by 4  DigitalFilter=No filtering  PulseInput=TTL level input  Direction=Down in the clockwise direction/Up in the counterclockwise direction  InitialValue=counter_offset_init  LoadInitialValue=on  SampleTime=dt  PciSlot=[1,13]  StartMethod=Model Start  StopMethod=Model Terminate  ZeroClearRising=off  ZeroClearFalling=off  ZeroClearMatch0=off  ZeroClearMatch1=off  PresetRising=off  PresetFalling=off  PresetMatch0=off  PresetMatch1=off  PresetValue=0  Match0Value=0  Match1Value=0  OutputSignalMatch0=off  OutputSignalMatch1=off  OutputSignalAbnormal=off  OutputSignalDigitalFilter=off  OutputSignalAlarm=off  OneShotDuration=10 microseconds  IndexEnable=Disable  IndexLogic=Positive (Active High)  EnableDigitalInput=off  EnableDigitalOutput=off  DigitalOutputInitialValue=None  DigitalOutputFinalValue=None
  Out1 : Outport
  wires:
  enc 1/1 -> Mux/1
  enc 2/1 -> Mux/2
  enc 3/1 -> Mux/3
  enc 4/1 -> Mux/4
  enc 5/1 -> Mux/5
  enc 6/1 -> Mux/6
  enc 7/1 -> Mux/7
  enc 8/1 -> Mux/8
  Mux/1 -> Out1/1

== system irep_single_axis/In-Vivo System/CONTEC CARDS/Level 2 ==
  Mux : Mux  Inputs=8
  enc 1 : xpcconteclib/Incremental Encoder/CNT32-8M(PCI)   Channel=1  OperationMode=2-phase Input Synchronous Clear Multiply by 4  DigitalFilter=No filtering  PulseInput=TTL level input  Direction=Down in the clockwise direction/Up in the counterclockwise direction  InitialValue=counter_offset_init  LoadInitialValue=on  SampleTime=dt  PciSlot=[2,8]  StartMethod=Model Start  StopMethod=Model Terminate  ZeroClearRising=off  ZeroClearFalling=off  ZeroClearMatch0=off  ZeroClearMatch1=off  PresetRising=on  PresetFalling=off  PresetMatch0=off  PresetMatch1=off  PresetValue=0  Match0Value=0  Match1Value=0  OutputSignalMatch0=off  OutputSignalMatch1=off  OutputSignalAbnormal=off  OutputSignalDigitalFilter=off  OutputSignalAlarm=off  OneShotDuration=10 microseconds  IndexEnable=Disable  IndexLogic=Positive (Active High)  EnableDigitalInput=off  EnableDigitalOutput=off  DigitalOutputInitialValue=None  DigitalOutputFinalValue=None
  enc 2 : xpcconteclib/Incremental Encoder/CNT32-8M(PCI)   Channel=2  OperationMode=2-phase Input Synchronous Clear Multiply by 4  DigitalFilter=No filtering  PulseInput=TTL level input  Direction=Up in the clockwise direction/Down in the counterclockwise direction  InitialValue=counter_offset_init  LoadInitialValue=on  SampleTime=dt  PciSlot=[2,8]  StartMethod=Model Start  StopMethod=Model Terminate  ZeroClearRising=off  ZeroClearFalling=off  ZeroClearMatch0=off  ZeroClearMatch1=off  PresetRising=off  PresetFalling=off  PresetMatch0=off  PresetMatch1=off  PresetValue=0  Match0Value=0  Match1Value=0  OutputSignalMatch0=off  OutputSignalMatch1=off  OutputSignalAbnormal=off  OutputSignalDigitalFilter=off  OutputSignalAlarm=off  OneShotDuration=10 microseconds  IndexEnable=Disable  IndexLogic=Positive (Active High)  EnableDigitalInput=off  EnableDigitalOutput=off  DigitalOutputInitialValue=None  DigitalOutputFinalValue=None
  enc 3 : xpcconteclib/Incremental Encoder/CNT32-8M(PCI)   Channel=3  OperationMode=2-phase Input Synchronous Clear Multiply by 4  DigitalFilter=No filtering  PulseInput=TTL level input  Direction=Up in the clockwise direction/Down in the counterclockwise direction  InitialValue=counter_offset_init  LoadInitialValue=on  SampleTime=dt  PciSlot=[2,8]  StartMethod=Model Start  StopMethod=Model Terminate  ZeroClearRising=off  ZeroClearFalling=off  ZeroClearMatch0=off  ZeroClearMatch1=off  PresetRising=off  PresetFalling=off  PresetMatch0=off  PresetMatch1=off  PresetValue=0  Match0Value=0  Match1Value=0  OutputSignalMatch0=off  OutputSignalMatch1=off  OutputSignalAbnormal=off  OutputSignalDigitalFilter=off  OutputSignalAlarm=off  OneShotDuration=10 microseconds  IndexEnable=Disable  IndexLogic=Positive (Active High)  EnableDigitalInput=off  EnableDigitalOutput=off  DigitalOutputInitialValue=None  DigitalOutputFinalValue=None
  enc 4 : xpcconteclib/Incremental Encoder/CNT32-8M(PCI)   Channel=4  OperationMode=2-phase Input Synchronous Clear Multiply by 4  DigitalFilter=No filtering  PulseInput=TTL level input  Direction=Up in the clockwise direction/Down in the counterclockwise direction  InitialValue=counter_offset_init  LoadInitialValue=on  SampleTime=dt  PciSlot=[2,8]  StartMethod=Model Start  StopMethod=Model Terminate  ZeroClearRising=off  ZeroClearFalling=off  ZeroClearMatch0=off  ZeroClearMatch1=off  PresetRising=off  PresetFalling=off  PresetMatch0=off  PresetMatch1=off  PresetValue=0  Match0Value=0  Match1Value=0  OutputSignalMatch0=off  OutputSignalMatch1=off  OutputSignalAbnormal=off  OutputSignalDigitalFilter=off  OutputSignalAlarm=off  OneShotDuration=10 microseconds  IndexEnable=Disable  IndexLogic=Positive (Active High)  EnableDigitalInput=off  EnableDigitalOutput=off  DigitalOutputInitialValue=None  DigitalOutputFinalValue=None
  enc 5 : xpcconteclib/Incremental Encoder/CNT32-8M(PCI)   Channel=5  OperationMode=2-phase Input Synchronous Clear Multiply by 4  DigitalFilter=No filtering  PulseInput=TTL level input  Direction=Up in the clockwise direction/Down in the counterclockwise direction  InitialValue=counter_offset_init  LoadInitialValue=on  SampleTime=dt  PciSlot=[2,8]  StartMethod=Model Start  StopMethod=Model Terminate  ZeroClearRising=off  ZeroClearFalling=off  ZeroClearMatch0=off  ZeroClearMatch1=off  PresetRising=off  PresetFalling=off  PresetMatch0=off  PresetMatch1=off  PresetValue=0  Match0Value=0  Match1Value=0  OutputSignalMatch0=off  OutputSignalMatch1=off  OutputSignalAbnormal=off  OutputSignalDigitalFilter=off  OutputSignalAlarm=off  OneShotDuration=10 microseconds  IndexEnable=Disable  IndexLogic=Positive (Active High)  EnableDigitalInput=off  EnableDigitalOutput=off  DigitalOutputInitialValue=None  DigitalOutputFinalValue=None
  enc 6 : xpcconteclib/Incremental Encoder/CNT32-8M(PCI)   Channel=6  OperationMode=2-phase Input Synchronous Clear Multiply by 4  DigitalFilter=No filtering  PulseInput=TTL level input  Direction=Down in the clockwise direction/Up in the counterclockwise direction  InitialValue=counter_offset_init  LoadInitialValue=on  SampleTime=dt  PciSlot=[2,8]  StartMethod=Model Start  StopMethod=Model Terminate  ZeroClearRising=off  ZeroClearFalling=off  ZeroClearMatch0=off  ZeroClearMatch1=off  PresetRising=off  PresetFalling=off  PresetMatch0=off  PresetMatch1=off  PresetValue=0  Match0Value=0  Match1Value=0  OutputSignalMatch0=off  OutputSignalMatch1=off  OutputSignalAbnormal=off  OutputSignalDigitalFilter=off  OutputSignalAlarm=off  OneShotDuration=10 microseconds  IndexEnable=Disable  IndexLogic=Positive (Active High)  EnableDigitalInput=off  EnableDigitalOutput=off  DigitalOutputInitialValue=None  DigitalOutputFinalValue=None
  enc 7 : xpcconteclib/Incremental Encoder/CNT32-8M(PCI)   Channel=7  OperationMode=2-phase Input Synchronous Clear Multiply by 4  DigitalFilter=No filtering  PulseInput=TTL level input  Direction=Down in the clockwise direction/Up in the counterclockwise direction  InitialValue=counter_offset_init  LoadInitialValue=on  SampleTime=dt  PciSlot=[2,8]  StartMethod=Model Start  StopMethod=Model Terminate  ZeroClearRising=off  ZeroClearFalling=off  ZeroClearMatch0=off  ZeroClearMatch1=off  PresetRising=off  PresetFalling=off  PresetMatch0=off  PresetMatch1=off  PresetValue=0  Match0Value=0  Match1Value=0  OutputSignalMatch0=off  OutputSignalMatch1=off  OutputSignalAbnormal=off  OutputSignalDigitalFilter=off  OutputSignalAlarm=off  OneShotDuration=10 microseconds  IndexEnable=Disable  IndexLogic=Positive (Active High)  EnableDigitalInput=off  EnableDigitalOutput=off  DigitalOutputInitialValue=None  DigitalOutputFinalValue=None
  enc 8 : xpcconteclib/Incremental Encoder/CNT32-8M(PCI)   Channel=8  OperationMode=2-phase Input Synchronous Clear Multiply by 4  DigitalFilter=No filtering  PulseInput=TTL level input  Direction=Down in the clockwise direction/Up in the counterclockwise direction  InitialValue=counter_offset_init  LoadInitialValue=on  SampleTime=dt  PciSlot=[2,8]  StartMethod=Model Start  StopMethod=Model Terminate  ZeroClearRising=off  ZeroClearFalling=off  ZeroClearMatch0=off  ZeroClearMatch1=off  PresetRising=off  PresetFalling=off  PresetMatch0=off  PresetMatch1=off  PresetValue=0  Match0Value=0  Match1Value=0  OutputSignalMatch0=off  OutputSignalMatch1=off  OutputSignalAbnormal=off  OutputSignalDigitalFilter=off  OutputSignalAlarm=off  OneShotDuration=10 microseconds  IndexEnable=Disable  IndexLogic=Positive (Active High)  EnableDigitalInput=off  EnableDigitalOutput=off  DigitalOutputInitialValue=None  DigitalOutputFinalValue=None
  Out1 : Outport
  wires:
  enc 1/1 -> Mux/1
  enc 2/1 -> Mux/2
  enc 3/1 -> Mux/3
  enc 4/1 -> Mux/4
  enc 5/1 -> Mux/5
  enc 6/1 -> Mux/6
  enc 7/1 -> Mux/7
  enc 8/1 -> Mux/8
  Mux/1 -> Out1/1
